simulink model "Sentinel_model_1elem"  (R2017b)
settings: Solver=VariableStepAuto  StartTime=0.0  StopTime=10.0  RelTol=1e-3
values from neighbouring files (symbols this model uses):
  Jzz_SA = 212    [Three_panels_1elem.m]
undefined symbols (not defined in the file or in its folder): M_SA
undefined symbols (not defined in the file): C_xy_1, C_xy_2, C_xy_3, E, ind_1, ind_2, ind_3, lx_1, lx_2, lx_3, ly_1, ly_2, ly_3, ni, P_xy_1, P_xy_2, P_xy_3, rho
libraries: cstblocks x3
settings Model: Creator=a.brugnoli  LastModifiedBy=a.brugnoli
settings DebuggingCC: InitInArrayFormatMsg=none

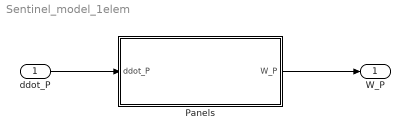
== system Sentinel_model_1elem ==
  ddot_P : Inport  PortDimensions=6
  Panels : Subsystem
  W_P : Outport
  wires:
  ddot_P/1 -> Panels/1(ddot_P)
  Panels/1(W_P) -> W_P/1

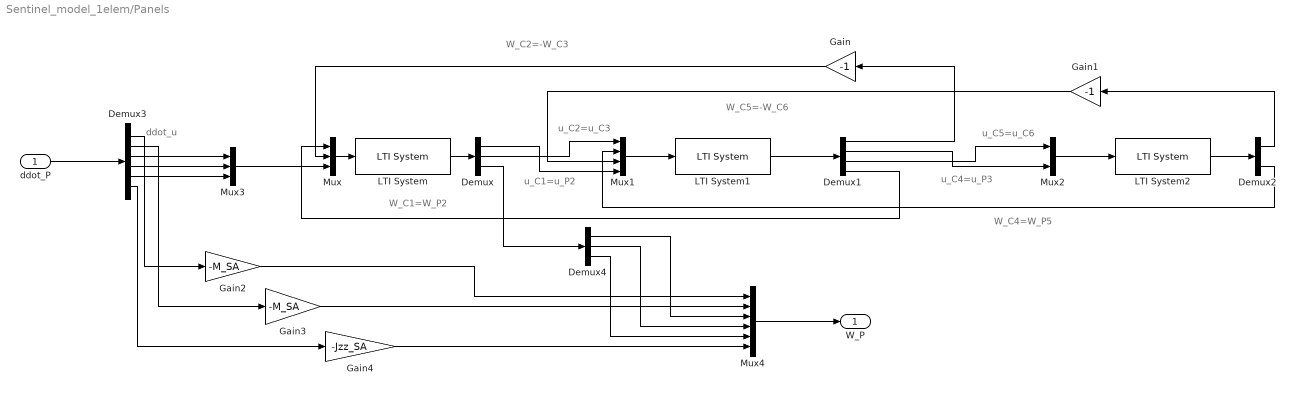
== system Sentinel_model_1elem/Panels ==
  note: ddot_u
  note: W_C2=-W_C3
  note: u_C1=u_P2
  note: u_C4=u_P3
  note: u_C2=u_C3
  note: W_C1=W_P2
  note: W_C5=-W_C6
  note: W_C4=W_P5
  note: u_C5=u_C6
  ddot_P : Inport
  Demux : Demux  Outputs=[3 3 3]
  Demux1 : Demux  Outputs=[3 3 3 3]
  Demux2 : Demux  Outputs=[3 3]
  Demux3 : Demux  Outputs=6
  Demux4 : Demux  Outputs=3
  Gain : Gain  Gain=-1
  Gain1 : Gain  Gain=-1
  Gain2 : Gain  Gain=-M_SA
  Gain3 : Gain  Gain=-M_SA
  Gain4 : Gain  Gain=-Jzz_SA
  LTI System : cstblocks/LTI System  sys=MFzTxTy  IC=[]  mask(LTI Block){lx=lx_1, ly=ly_1, t=t, rho=rho, E=E, ni=ni, P_xy=P_xy_1, C_xy=C_xy_1, ind=ind_1}
      mask prompts: lx "Horizontal length"; ly "Vertical length"; t "Thickness"; rho "Mass Density"; E "Young Modulus"; ni "Poisson ratio"; P_xy "Number of the parent node"; C_xy "Vector of children nodes numbers"; ind "Indexes of ports to be inverted (0 if no inversion is required)"
      mask init:
      | MFzTxTy = Kirchhoff_1elem(lx, ly, t, rho, E, ni, P_xy, C_xy);
      | if ind~=0
      |     MFzTxTy = invio(MFzTxTy, ind);
      | end
      mask Help:
      | [MtzRyRx] = NPort_KirchhoffTzRyRx(l1,l2,t,rho,E,ni,nx,ny,P_id,C_ids,xi)
      | Finite Element Model MtzRyRx (6x6) of a uniform Kirchhoff plate characterized by:
      |   * plate length along x: l1 (m),
      |   * plate length along y: l2 (m),
      |   * plate thikness along z: t (m),
      |   * mass density: rho  (Kg/m^3),
      |   * Young modulus: E (Pascal or N/m^2),
      |   * Poisson ratio: ni,
      |   * number of 4-node plate elements along x: nx,
      |   * number of 4-node plate elements along y: ny,
      |   * ID number of parent node P: P_id (see NOTE for nodal convention),
      |   * ID number of children nodes (vector): C_ids (see NOTE for nodal convention),
      |   * xi: arbitrary damping ratio for all flexible modes.
      | 
      |          ^ z    y
      |          |     /
      |          |    /             C (x=0, y=ly)
      |          |   -----------------------/
      |          |  /                  *   /
      |          | * P(xp = 0,yp)         /
      |          |/                      /
      |          .----------------------/----------> x
      |     (x=0, y=0)
      | 
      | 
      |   Only pure flexion in the plane (P,x,z) and torsion in the plane (P,y,z) are considered.
      | 
      |   The 3*(Number of Children + 1) inputs of MtzRyRx are:
      |      * the external force F_Cz (along z) and torques T_Cx (around x)
      |        and T_Cy (around y) applied to the plate at point C,
      |      * the linear ddot(z)_P (along z) and angular ddot(theta_x)_P
      |        (around x) and ddot(theta_y)_P (around y) accelerations at point P.
      |   The 3*(Number of Children + 1) outputs of M are:
      |      * the linear ddot(z)_C (along z) and angular ddot(theta_x)_C
      |        (around x) and ddot(theta_y)_C (around y) accelerations at point C,
      |      * the external force F_Pz (along z) and torques T_Px (around x)
      |        and T_Py (around y) applied to the plate at point P.
      | 
      |  NOTE: Example for a 4x5 elements plate: global node convention
      | 
      |  25----26----27----28----29----30
      |   |   16 |    17 |     18 |   19 |    20 |
      |  19----20----21----22----23----24
      |   | 11   |    12 |  13   |  14   |  15   |
      |  13----14----15----16----17----18
      |   | 6      |  7    |  8     |  9     |   10  |
      |   7----8-----9-----10----11----12
      |   |   1   |   2   |   3   |    4   |    5    |
      |   1----2-----3-----4-----5-----6
  LTI System1 : cstblocks/LTI System  sys=MFzTxTy  IC=[]  mask(LTI Block){lx=lx_2, ly=ly_2, t=t, rho=rho, E=E, ni=ni, P_xy=P_xy_2, C_xy=C_xy_2, ind=ind_2}
      mask prompts: lx "Horizontal length"; ly "Vertical length"; t "Thickness"; rho "Mass Density"; E "Young Modulus"; ni "Poisson ratio"; P_xy "Number of the parent node"; C_xy "Vector of children nodes numbers"; ind "Indexes of ports to be inverted (0 if no inversion is required)"
      mask init:
      | MFzTxTy = Kirchhoff_1elem(lx, ly, t, rho, E, ni, P_xy, C_xy);
      | if ind~=0
      |     MFzTxTy = invio(MFzTxTy, ind);
      | end
      mask Help:
      | [MtzRyRx] = NPort_KirchhoffTzRyRx(l1,l2,t,rho,E,ni,nx,ny,P_id,C_ids,xi)
      | Finite Element Model MtzRyRx (6x6) of a uniform Kirchhoff plate characterized by:
      |   * plate length along x: l1 (m),
      |   * plate length along y: l2 (m),
      |   * plate thikness along z: t (m),
      |   * mass density: rho  (Kg/m^3),
      |   * Young modulus: E (Pascal or N/m^2),
      |   * Poisson ratio: ni,
      |   * number of 4-node plate elements along x: nx,
      |   * number of 4-node plate elements along y: ny,
      |   * ID number of parent node P: P_id (see NOTE for nodal convention),
      |   * ID number of children nodes (vector): C_ids (see NOTE for nodal convention),
      |   * xi: arbitrary damping ratio for all flexible modes.
      | 
      |          ^ z    y
      |          |     /
      |          |    /             C (x=0, y=ly)
      |          |   -----------------------/
      |          |  /                  *   /
      |          | * P(xp = 0,yp)         /
      |          |/                      /
      |          .----------------------/----------> x
      |     (x=0, y=0)
      | 
      | 
      |   Only pure flexion in the plane (P,x,z) and torsion in the plane (P,y,z) are considered.
      | 
      |   The 3*(Number of Children + 1) inputs of MtzRyRx are:
      |      * the external force F_Cz (along z) and torques T_Cx (around x)
      |        and T_Cy (around y) applied to the plate at point C,
      |      * the linear ddot(z)_P (along z) and angular ddot(theta_x)_P
      |        (around x) and ddot(theta_y)_P (around y) accelerations at point P.
      |   The 3*(Number of Children + 1) outputs of M are:
      |      * the linear ddot(z)_C (along z) and angular ddot(theta_x)_C
      |        (around x) and ddot(theta_y)_C (around y) accelerations at point C,
      |      * the external force F_Pz (along z) and torques T_Px (around x)
      |        and T_Py (around y) applied to the plate at point P.
      | 
      |  NOTE: Example for a 4x5 elements plate: global node convention
      | 
      |  25----26----27----28----29----30
      |   |   16 |    17 |     18 |   19 |    20 |
      |  19----20----21----22----23----24
      |   | 11   |    12 |  13   |  14   |  15   |
      |  13----14----15----16----17----18
      |   | 6      |  7    |  8     |  9     |   10  |
      |   7----8-----9-----10----11----12
      |   |   1   |   2   |   3   |    4   |    5    |
      |   1----2-----3-----4-----5-----6
  LTI System2 : cstblocks/LTI System  sys=MFzTxTy  IC=[]  mask(LTI Block){lx=lx_3, ly=ly_3, t=t, rho=rho, E=E, ni=ni, P_xy=P_xy_3, C_xy=C_xy_3, ind=ind_3}
      mask prompts: lx "Horizontal length"; ly "Vertical length"; t "Thickness"; rho "Mass Density"; E "Young Modulus"; ni "Poisson ratio"; P_xy "Number of the parent node"; C_xy "Vector of children nodes numbers"; ind "Indexes of ports to be inverted (0 if no inversion is required)"
      mask init:
      | MFzTxTy = Kirchhoff_1elem(lx, ly, t, rho, E, ni, P_xy, C_xy);
      | if ind~=0
      |     MFzTxTy = invio(MFzTxTy, ind);
      | end
      mask Help:
      | [MtzRyRx] = NPort_KirchhoffTzRyRx(l1,l2,t,rho,E,ni,nx,ny,P_id,C_ids,xi)
      | Finite Element Model MtzRyRx (6x6) of a uniform Kirchhoff plate characterized by:
      |   * plate length along x: l1 (m),
      |   * plate length along y: l2 (m),
      |   * plate thikness along z: t (m),
      |   * mass density: rho  (Kg/m^3),
      |   * Young modulus: E (Pascal or N/m^2),
      |   * Poisson ratio: ni,
      |   * number of 4-node plate elements along x: nx,
      |   * number of 4-node plate elements along y: ny,
      |   * ID number of parent node P: P_id (see NOTE for nodal convention),
      |   * ID number of children nodes (vector): C_ids (see NOTE for nodal convention),
      |   * xi: arbitrary damping ratio for all flexible modes.
      | 
      |          ^ z    y
      |          |     /
      |          |    /             C (x=0, y=ly)
      |          |   -----------------------/
      |          |  /                  *   /
      |          | * P(xp = 0,yp)         /
      |          |/                      /
      |          .----------------------/----------> x
      |     (x=0, y=0)
      | 
      | 
      |   Only pure flexion in the plane (P,x,z) and torsion in the plane (P,y,z) are considered.
      | 
      |   The 3*(Number of Children + 1) inputs of MtzRyRx are:
      |      * the external force F_Cz (along z) and torques T_Cx (around x)
      |        and T_Cy (around y) applied to the plate at point C,
      |      * the linear ddot(z)_P (along z) and angular ddot(theta_x)_P
      |        (around x) and ddot(theta_y)_P (around y) accelerations at point P.
      |   The 3*(Number of Children + 1) outputs of M are:
      |      * the linear ddot(z)_C (along z) and angular ddot(theta_x)_C
      |        (around x) and ddot(theta_y)_C (around y) accelerations at point C,
      |      * the external force F_Pz (along z) and torques T_Px (around x)
      |        and T_Py (around y) applied to the plate at point P.
      | 
      |  NOTE: Example for a 4x5 elements plate: global node convention
      | 
      |  25----26----27----28----29----30
      |   |   16 |    17 |     18 |   19 |    20 |
      |  19----20----21----22----23----24
      |   | 11   |    12 |  13   |  14   |  15   |
      |  13----14----15----16----17----18
      |   | 6      |  7    |  8     |  9     |   10  |
      |   7----8-----9-----10----11----12
      |   |   1   |   2   |   3   |    4   |    5    |
      |   1----2-----3-----4-----5-----6
  Mux : Mux  Inputs=3
  Mux1 : Mux
  Mux2 : Mux  Inputs=2
  Mux3 : Mux  Inputs=3
  Mux4 : Mux  Inputs=6
  W_P : Outport
  wires:
  Mux3/1 -> Mux/3
  Gain1/1 -> Mux1/3
  Demux1/3 -> Mux2/1
  Mux2/1 -> LTI System2/1
  LTI System2/1 -> Demux2/1
  Demux1/1 -> Gain/1
  Demux1/2 -> Mux2/2
  Mux1/1 -> LTI System1/1
  Demux4/1 -> Mux4/3
  Gain4/1 -> Mux4/6
  ddot_P/1 -> Demux3/1
  Gain2/1 -> Mux4/1
  Demux4/3 -> Mux4/5
  Demux4/2 -> Mux4/4
  Demux3/5 -> Mux3/3
  Demux3/3 -> Mux3/1
  Demux3/1 -> Gain2/1
  Demux3/4 -> Mux3/2
  Mux4/1 -> W_P/1
  Demux3/2 -> Gain3/1
  Demux3/6 -> Gain4/1
  Gain3/1 -> Mux4/2
  Demux1/4 -> Mux/1
  Demux/3 -> Demux4/1
  Demux2/2 -> Mux1/2
  Gain/1 -> Mux/2
  Demux/2 -> Mux1/1
  Mux/1 -> LTI System/1
  LTI System1/1 -> Demux1/1
  Demux2/1 -> Gain1/1
  Demux/1 -> Mux1/4
  LTI System/1 -> Demux/1
